simulink model "exc2"  (R2024b)
settings: Solver=VariableStepAuto  StartTime=0.0  StopTime=10.0  RelTol=1e-3
settings Model: Creator=ramse  LastModifiedBy=ramse

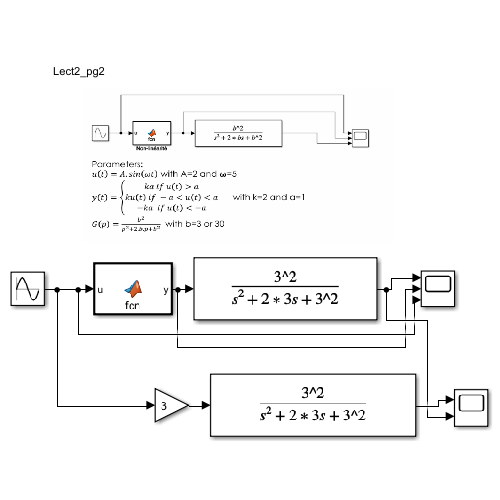
[thumbnail: Simulink's stored preview of the top-level diagram]
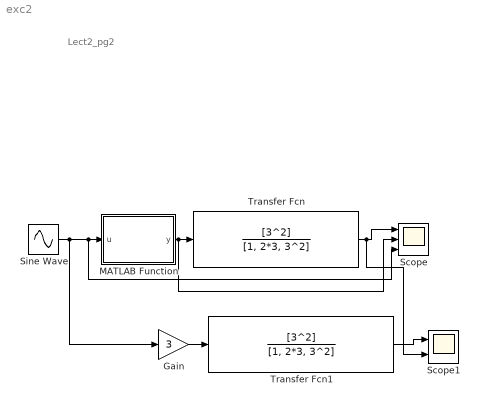
== system exc2 ==
  note: Lect2_pg2
  Gain : Gain  Gain=3
  MATLAB Function : MATLAB Function  TreatAsAtomicUnit=on
  Scope : Scope  NumInputPorts=3
  Scope1 : Scope  NumInputPorts=2
  Sine Wave : Sin  Frequency=5  SampleTime=0
  Transfer Fcn : TransferFcn  Numerator=[3^2]  Denominator=[1, 2*3, 3^2]
  Transfer Fcn1 : TransferFcn  Numerator=[3^2]  Denominator=[1, 2*3, 3^2]
  wires:
  MATLAB Function/1(y) -> Scope/2, Transfer Fcn/1
  Transfer Fcn/1 -> Scope1/2, Scope/1
  Sine Wave/1 -> Gain/1, Scope/3, MATLAB Function/1(u)
  Gain/1 -> Transfer Fcn1/1
  Transfer Fcn1/1 -> Scope1/1

== matlab function exc2/MATLAB Function ==
  data: u input; y output
function y = fcn(u)
k=2;
a=1;
if u>a
    y=k*a;
elseif (-a<u) && (u<a)
    y=k*u;
else
    y=-k*a;
end
